simulink model "Q_2_Numerical_Simulations"  (R2024b)
settings: Solver=ode45  StartTime=0.0  StopTime=100.0  FixedStep=0.001  RelTol=1e-3
InitFcn:
  | load_params_inertial_case
  | PID_calculations
values from neighbouring files (symbols this model uses):
  J_eq = mot.J + (3*gbox.J72 + mld.J) / gbox.N^2    [PID_calculations.m]
  K_D = K_P * T_D    [PID_calculations.m]
  K_I = K_P / T_I    [PID_calculations.m]
  K_P = DeltaK * cos(DeltaPhi)    [PID_calculations.m]
  R_eq = mot.Ra + mot.Rs    [PID_calculations.m]
  T_L = 5 * w_gc    [PID_calculations.m]
undefined symbols (not defined in the file or in its folder): B_eq_model, drv, gbox, mot, rads2rpm, sens, t_sf_model
libraries: slpidlib x1
settings Model: Creator=JS  LastModifiedBy=JS
settings SolverCC: ZeroCrossAlgorithm=Adaptive
settings DebuggingCC: IgnoredZcDiagnostic=none

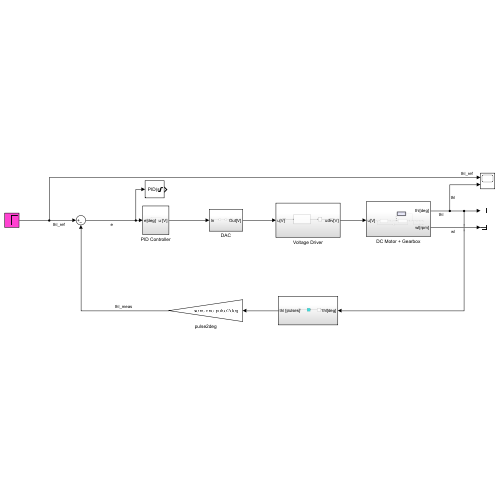
[thumbnail: Simulink's stored preview of the top-level diagram]
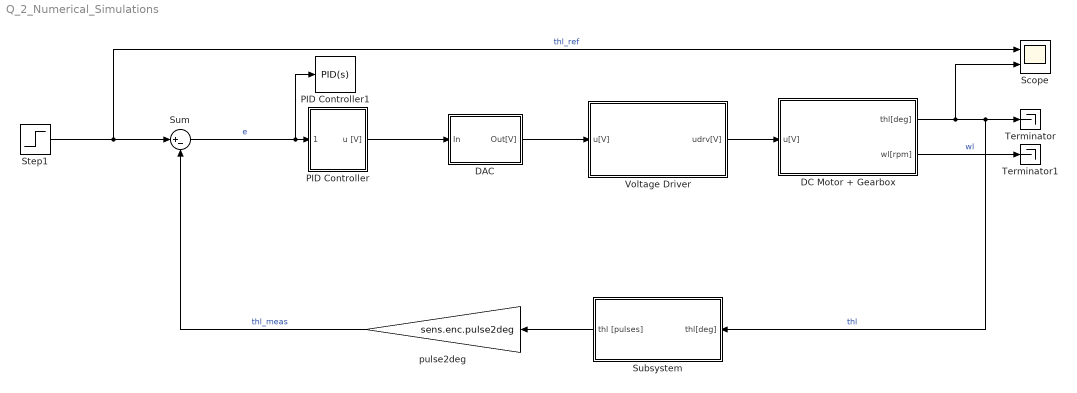
== system Q_2_Numerical_Simulations ==
  DAC : Subsystem
  DC Motor + Gearbox : Subsystem
  PID Controller : Subsystem
  PID Controller1 : slpidlib/PID Controller  Controller=PID  Form=Parallel  TimeDomain=Continuous-time  UseExternalTs=off  SampleTime=-1  IntegratorMethod=Forward Euler  FilterMethod=Forward Euler  ControllerParametersSource=internal  P=8.5  I=7  UseKiTs=off  D=0.06  UseExternalDerivativeSource=off  N=55467.0568791698  UseFilter=on  TunerSelectOption=Transfer Function Based (PID Tuner App)  InitialConditionSource=internal  InitialConditionForIntegrator=0  InitialConditionForFilter=0  DifferentiatorICPrevScaledInput=0  ExternalReset=none  TrackingMode=off  Kt=1  LimitOutput=on  SatLimitsSource=internal  UpperSaturationLimit=10  LowerSaturationLimit=-10  LinearizeAsGain=on  AntiWindupMode=none  Kb=1  LimitIntegrator=off  UpperIntegratorSaturationLimit=inf  LowerIntegratorSaturationLimit=-inf  POutMin=[]  POutMax=[]  IOutMin=[]  IOutMax=[]  DOutMin=[]  DOutMax=[]  NOutMin=[]  NOutMax=[]  SumOutMin=[]  SumOutMax=[]  SaturationOutMin=[]  SaturationOutMax=[]  PParamMin=[]  PParamMax=[]  IParamMin=[]  IParamMax=[]  DParamMin=[]  DParamMax=[]  NParamMin=[]  NParamMax=[]  KbParamMin=[]  KbParamMax=[]  KtParamMin=[]  KtParamMax=[]  KbOutMin=[]  KbOutMax=[]  KtOutMin=[]  KtOutMax=[]  IntegratorOutMin=[]  IntegratorOutMax=[]  FilterOutMin=[]  FilterOutMax=[]  SumI1OutMin=[]  SumI1OutMax=[]  SumI2OutMin=[]  SumI2OutMax=[]  SumI3OutMin=[]  SumI3OutMax=[]  SumI4OutMin=[]  SumI4OutMax=[]  SumDOutMin=[]  SumDOutMax=[]  DifferentiatorOutMin=[]  DifferentiatorOutMax=[]  FilterDiffOutCoefMin=[]  FilterDiffOutCoefMax=[]  ReciprocalOutMin=[]  ReciprocalOutMax=[]  SumDenOutMin=[]  SumDenOutMax=[]  SumNumOutMin=[]  SumNumOutMax=[]  DivideOutMin=[]  DivideOutMax=[]  UdiffTsProdOutMin=[]  UdiffTsProdOutMax=[]  NTsProdOutMin=[]  NTsProdOutMax=[]  UintegralTsProdOutMin=[]  UintegralTsProdOutMax=[]  UngainTsProdOutMin=[]  UngainTsProdOutMax=[]  ClampingZeroOutDataTypeStr=Inherit: Inherit via back propagation  ClampingZeroOutMin=[]  ClampingZeroOutMax=[]  FilterDenConstantOutDataTypeStr=Inherit: Inherit via back propagation  FilterDenConstantOutMin=[]  FilterDenConstantOutMax=[]  PCopyOutDataTypeStr=Inherit: Inherit via back propagation  PCopyOutMin=[]  PCopyOutMax=[]  NCopyOutDataTypeStr=Inherit: Inherit via back propagation  NCopyOutMin=[]  NCopyOutMax=[]  IntegratorContinuousStateAttributes=''  IntegratorStateMustResolveToSignalObject=off  IntegratorRTWStateStorageClass=Auto  FilterContinuousStateAttributes=''  FilterStateMustResolveToSignalObject=off  FilterRTWStateStorageClass=Auto  ParallelPVariant=InternalParameters  IdealPVariant=Disabled  IVariant=InternalParameters  DVariant=InternalParameters  IntegratorVariant=Continuous  SatVariant=Enabled  AWVariant=Passthrough  PCopyVariant=Disabled  TRVariant=Disabled  FdbkBlocksVariant=Forward  IdealPFdbkVariant=Disabled  SatFdbkVariant=Disabled  DerivativeFilterVariant=ContFilter  NVariant=InternalParameters  NCopyVariant=Disabled  FilterICVariant=InternalICsFilter  IntegratorICVariant=InternalICs  ExternalResetVariant=Disabled  TRSumVariant=Passthrough  SumFdbkVariant=Disabled  SumVariant=Sum_PID  TsampFilterVariant=InternalTs  TsampNgainVariant=Passthrough  TsampIntegralVariant=Disabled_SignalSpec  ExternalSaturationOutDataTypeStr=Inherit: Same as second input  DerivativeSourceVariant=ErrorSignal  PreIntVariant=InternalPreInt
  Scope : Scope  NumInputPorts=2
  Step1 : Step  Time=5  After=360  SampleTime=0
  Subsystem : Subsystem
  Sum : Sum  Inputs=|+-
  Terminator : Terminator
  Terminator1 : Terminator
  Voltage Driver : Subsystem
  pulse2deg : Gain  Gain=sens.enc.pulse2deg
  wires:
  Voltage Driver/1(udrv[V]) -> DC Motor + Gearbox/1(u[V])
  DC Motor + Gearbox/1(thl[deg]) -> Scope/2, Subsystem/1(thl[deg]), Terminator/1  "thl"
  DC Motor + Gearbox/2(wl[rpm]) -> Terminator1/1  "wl"
  DAC/1(Out[V]) -> Voltage Driver/1(u[V])
  Subsystem/1(thl [pulses]) -> pulse2deg/1
  pulse2deg/1 -> Sum/2  "thl_meas"
  Sum/1 -> PID Controller1/1, PID Controller/1(e[deg])  "e"
  Step1/1 -> Scope/1, Sum/1  "thl_ref"
  PID Controller/1(u [V]) -> DAC/1(In)

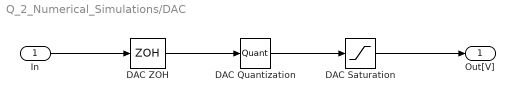
== system Q_2_Numerical_Simulations/DAC ==
  In : Inport
  DAC Quantization : Quantizer  QuantizationInterval=daq.dac.q
  DAC Saturation : Saturate  UpperLimit=10  LowerLimit=-10
  DAC ZOH : ZeroOrderHold  SampleTime=0.001
  Out[V] : Outport
  wires:
  DAC Saturation/1 -> Out[V]/1
  In/1 -> DAC ZOH/1
  DAC ZOH/1 -> DAC Quantization/1
  DAC Quantization/1 -> DAC Saturation/1

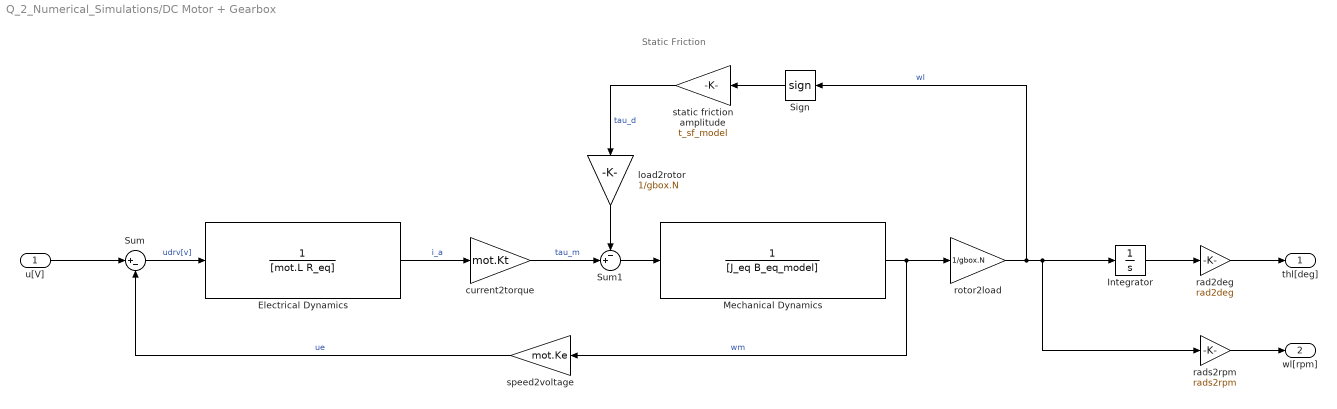
== system Q_2_Numerical_Simulations/DC Motor + Gearbox ==
  note: Static Friction
  u[V] : Inport
  Electrical Dynamics : TransferFcn  Denominator=[mot.L R_eq]
  Integrator : Integrator
  Mechanical Dynamics : TransferFcn  Denominator=[J_eq B_eq_model]
  Sign : Signum  ZeroCross=off
  Sum : Sum  Inputs=|+-
  Sum1 : Sum  Inputs=-+|
  current2torque : Gain  Gain=mot.Kt
  load2rotor : Gain  Gain=1/gbox.N
  rad2deg : Gain  Gain=rad2deg
  rads2rpm : Gain  Gain=rads2rpm
  rotor2load : Gain  Gain=1/gbox.N
  speed2voltage : Gain  Gain=mot.Ke
  static friction amplitude : Gain  Gain=t_sf_model
  thl[deg] : Outport
  wl[rpm] : Outport  Port=2
  wires:
  Integrator/1 -> rad2deg/1
  Mechanical Dynamics/1 -> speed2voltage/1, rotor2load/1  "wm"
  current2torque/1 -> Sum1/2  "tau_m"
  rotor2load/1 -> Sign/1, rads2rpm/1, Integrator/1  "wl"
  u[V]/1 -> Sum/1
  Electrical Dynamics/1 -> current2torque/1  "i_a"
  rad2deg/1 -> thl[deg]/1
  Sum/1 -> Electrical Dynamics/1  "udrv[v]"
  Sum1/1 -> Mechanical Dynamics/1
  rads2rpm/1 -> wl[rpm]/1
  Sign/1 -> static friction amplitude/1
  static friction amplitude/1 -> load2rotor/1  "tau_d"
  speed2voltage/1 -> Sum/2  "ue"
  load2rotor/1 -> Sum1/1

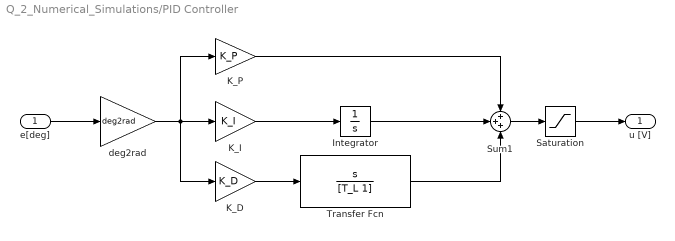
== system Q_2_Numerical_Simulations/PID Controller ==
  e[deg] : Inport
  Integrator : Integrator  ZeroCross=off
  K_D : Gain  Gain=K_D
  K_I : Gain  Gain=K_I
  K_P : Gain  Gain=K_P
  Saturation : Saturate  UpperLimit=10  LowerLimit=-10
  Sum1 : Sum  Inputs=+++
  Transfer Fcn : TransferFcn  Numerator=[1 0]  Denominator=[T_L 1]
  deg2rad : Gain  Gain=deg2rad
  u [V] : Outport
  wires:
  Sum1/1 -> Saturation/1
  deg2rad/1 -> K_P/1, K_D/1, K_I/1
  e[deg]/1 -> deg2rad/1
  K_D/1 -> Transfer Fcn/1
  Integrator/1 -> Sum1/2
  Saturation/1 -> u [V]/1
  K_I/1 -> Integrator/1
  Transfer Fcn/1 -> Sum1/3
  K_P/1 -> Sum1/1

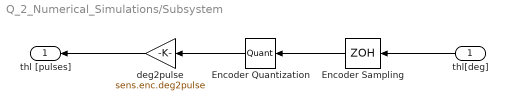
== system Q_2_Numerical_Simulations/Subsystem ==
  thl[deg] : Inport
  Encoder Quantization : Quantizer  QuantizationInterval=enc.q_all
  Encoder Sampling : ZeroOrderHold  SampleTime=0.001
  deg2pulse : Gain  Gain=sens.enc.deg2pulse
  thl [pulses] : Outport
  wires:
  thl[deg]/1 -> Encoder Sampling/1
  Encoder Quantization/1 -> deg2pulse/1
  Encoder Sampling/1 -> Encoder Quantization/1
  deg2pulse/1 -> thl [pulses]/1

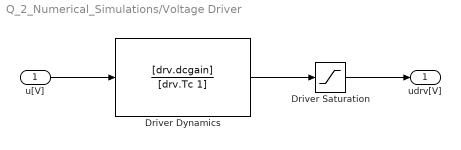
== system Q_2_Numerical_Simulations/Voltage Driver ==
  u[V] : Inport
  Driver Dynamics : TransferFcn  Numerator=[drv.dcgain]  Denominator=[drv.Tc 1]
  Driver Saturation : Saturate  UpperLimit=12  LowerLimit=-12
  udrv[V] : Outport
  wires:
  Driver Dynamics/1 -> Driver Saturation/1
  u[V]/1 -> Driver Dynamics/1
  Driver Saturation/1 -> udrv[V]/1
